simulink model "propcontroller"  (R2021b)
settings: Solver=VariableStepAuto  StartTime=0.0  StopTime=80  RelTol=1e-3
settings Model: Creator=mluser  LastModifiedBy=mluser

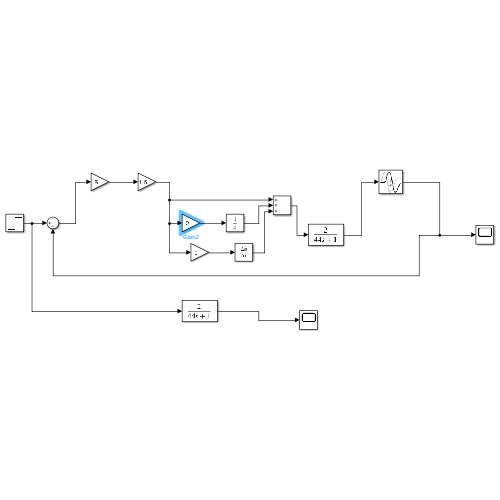
[thumbnail: Simulink's stored preview of the top-level diagram]
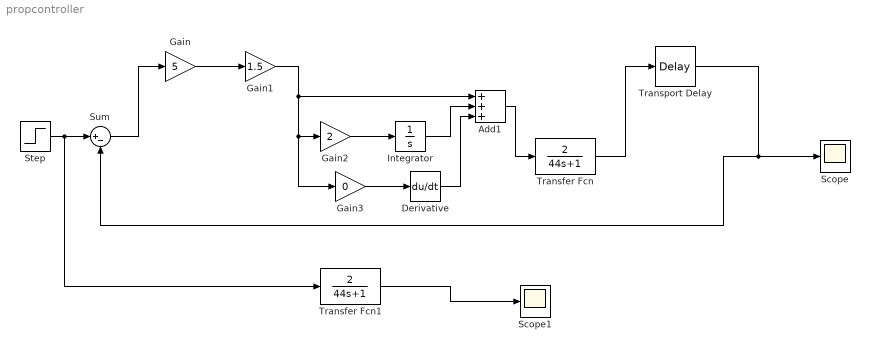
== system propcontroller ==
  Add1 : Sum  Inputs=+++
  Derivative : Derivative
  Gain : Gain  Gain=5
  Gain1 : Gain  Gain=1.5
  Gain2 : Gain  Gain=2
  Gain3 : Gain  Gain=0
  Integrator : Integrator
  Scope : Scope
  Scope1 : Scope
  Step : Step  Before=1  SampleTime=0.0001
  Sum : Sum  Inputs=|+-
  Transfer Fcn : TransferFcn  Numerator=[2]  Denominator=[44 1]
  Transfer Fcn1 : TransferFcn  Numerator=[2]  Denominator=[44 1]
  Transport Delay : TransportDelay
  wires:
  Step/1 -> Transfer Fcn1/1, Sum/1
  Sum/1 -> Gain/1
  Gain1/1 -> Add1/1, Gain3/1, Gain2/1
  Integrator/1 -> Add1/2
  Derivative/1 -> Add1/3
  Gain2/1 -> Integrator/1
  Gain3/1 -> Derivative/1
  Gain/1 -> Gain1/1
  Add1/1 -> Transfer Fcn/1
  Transfer Fcn1/1 -> Scope1/1
  Transfer Fcn/1 -> Transport Delay/1
  Transport Delay/1 -> Sum/2, Scope/1
